simulink model "Prova_orbita"  (R2023b)
settings: Solver=ode3  StartTime=0.0  StopTime=T  FixedStep=0.1  RelTol=1e-3
values from neighbouring files (symbols this model uses):
  A_0 = [1 0 0; 0 1 0; 0 0 1]    [orbita.m]
  I = [Ix 0 0; 0 Iy 0; 0 0 Iz]    [orbita.m]    (also in reaction_wheels_code.m)
  I_inv = inv(I)    [orbita.m]    (also in reaction_wheels_code.m)
  M = 0    [orbita.m]    (also in reaction_wheels_code.m)
  mu_E = astroConstants(13)    [orbita.m]
  mu_S = astroConstants(4)    [orbita.m]
  omega_0 = [0.45 0.52 0.55]'    [orbita.m]    (also in reaction_wheels_code.m = [0 0 0]')
  rot = [0 0 Ir*omega_r0]'    [orbita.m]
undefined symbols (not defined in the file or in its folder): r0, r0_E, v0, v0_E
libraries: LibrarySAD x2
settings Model: Creator=valen  LastModifiedBy=valen

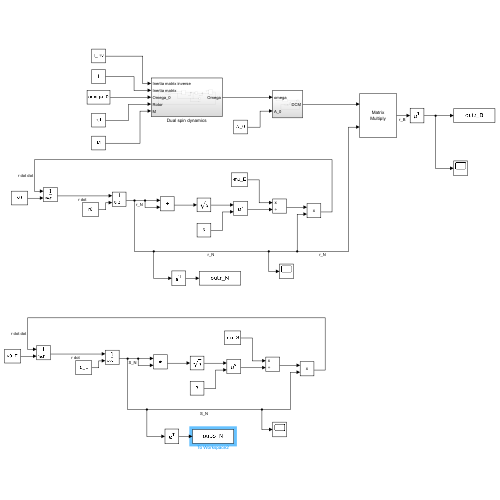
[thumbnail: Simulink's stored preview of the top-level diagram]
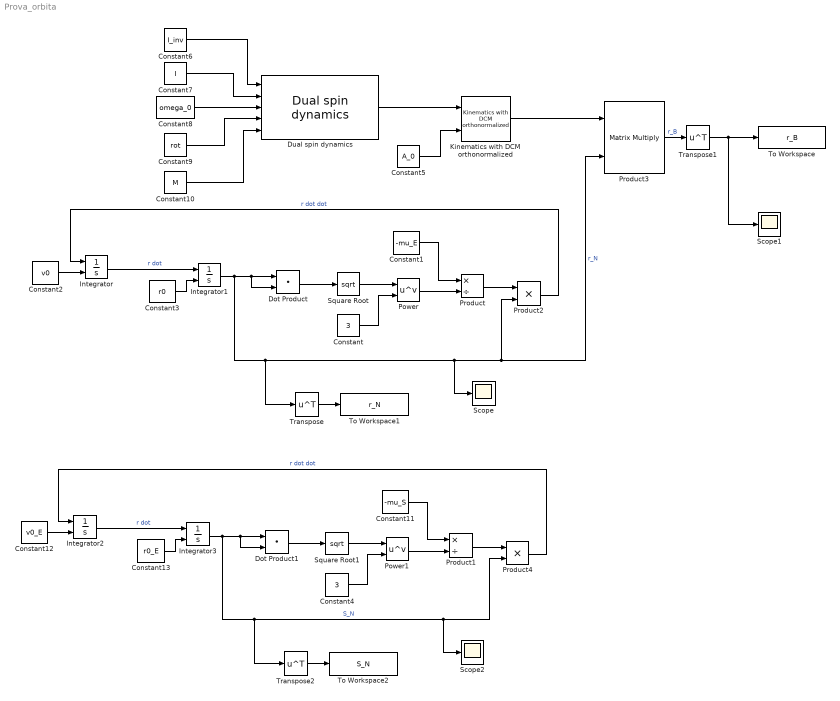
== system Prova_orbita ==
  Constant : Constant  Value=3
  Constant1 : Constant  Value=-mu_E  VectorParams1D=off
  Constant10 : Constant  Value=M  VectorParams1D=off
  Constant11 : Constant  Value=-mu_S  VectorParams1D=off
  Constant12 : Constant  Value=v0_E  VectorParams1D=off
  Constant13 : Constant  Value=r0_E  VectorParams1D=off
  Constant2 : Constant  Value=v0  VectorParams1D=off
  Constant3 : Constant  Value=r0  VectorParams1D=off
  Constant4 : Constant  Value=3
  Constant5 : Constant  Value=A_0  VectorParams1D=off
  Constant6 : Constant  Value=I_inv  VectorParams1D=off
  Constant7 : Constant  Value=I  VectorParams1D=off
  Constant8 : Constant  Value=omega_0  VectorParams1D=off
  Constant9 : Constant  Value=rot  VectorParams1D=off
  Dot Product : DotProduct  OutDataTypeStr=Inherit: Inherit via internal rule
  Dot Product1 : DotProduct  OutDataTypeStr=Inherit: Inherit via internal rule
  Dual spin dynamics : LibrarySAD/Dual spin dynamics  SystemSampleTime=-1  VariantActivationTime=update diagram  AllowFlexibleInterface=on  Latency=0  AutoFrameSizeCalculation=off
  Integrator{,1..3} (4 alike) : Integrator  InitialConditionSource=external
  Kinematics with DCM orthonormalized : LibrarySAD/Kinematics with DCM orthonormalized  SystemSampleTime=-1  VariantActivationTime=update diagram  AllowFlexibleInterface=on  Latency=0  AutoFrameSizeCalculation=off
  Power : Math  Operator=pow
  Power1 : Math  Operator=pow
  Product : Product  Inputs=*/
  Product1 : Product  Inputs=*/
  Product2 : Product
  Product3 : Product  Multiplication=Matrix(*)
  Product4 : Product
  Scope : Scope
  Scope1 : Scope
  Scope2 : Scope
  Square Root : Sqrt
  Square Root1 : Sqrt
  To Workspace : ToWorkspace  VariableName=r_B  SampleTime=-1
      settings: Save2DSignal=2-D array (concatenate along first dimension)
  To Workspace1 : ToWorkspace  VariableName=r_N  SampleTime=-1
      settings: Save2DSignal=2-D array (concatenate along first dimension)
  To Workspace2 : ToWorkspace  VariableName=S_N  SampleTime=-1
      settings: Save2DSignal=2-D array (concatenate along first dimension)
  Transpose : Math  Operator=transpose
  Transpose1 : Math  Operator=transpose
  Transpose2 : Math  Operator=transpose
  wires:
  Kinematics with DCM orthonormalized/1 -> Product3/1
  Product2/1 -> Integrator/1  "r dot dot"
  Constant5/1 -> Kinematics with DCM orthonormalized/2
  Constant8/1 -> Dual spin dynamics/3
  Constant7/1 -> Dual spin dynamics/2
  Constant9/1 -> Dual spin dynamics/4
  Constant10/1 -> Dual spin dynamics/5
  Dual spin dynamics/1 -> Kinematics with DCM orthonormalized/1
  Product3/1 -> Transpose1/1  "r_B"
  Constant6/1 -> Dual spin dynamics/1
  Constant2/1 -> Integrator/2
  Constant3/1 -> Integrator1/2
  Integrator/1 -> Integrator1/1  "r dot"
  Integrator1/1 -> Transpose/1, Product2/2, Product3/2, Scope/1, Dot Product/2, Dot Product/1  "r_N"
  Dot Product/1 -> Square Root/1
  Constant1/1 -> Product/1
  Product/1 -> Product2/1
  Transpose/1 -> To Workspace1/1
  Transpose1/1 -> Scope1/1, To Workspace/1
  Square Root/1 -> Power/1
  Constant/1 -> Power/2
  Power/1 -> Product/2
  Constant13/1 -> Integrator3/2
  Constant4/1 -> Power1/2
  Integrator2/1 -> Integrator3/1  "r dot"
  Square Root1/1 -> Power1/1
  Power1/1 -> Product1/2
  Constant12/1 -> Integrator2/2
  Constant11/1 -> Product1/1
  Transpose2/1 -> To Workspace2/1
  Dot Product1/1 -> Square Root1/1
  Integrator3/1 -> Transpose2/1, Product4/2, Scope2/1, Dot Product1/2, Dot Product1/1  "S_N"
  Product4/1 -> Integrator2/1  "r dot dot"
  Product1/1 -> Product4/1
